simulink model "Subsystem"  (R2020b)
settings: Solver=VariableStepAuto  StartTime=0.0  StopTime=10.0  RelTol=1e-3
settings Model: Creator=shivanshu shukla  LastModifiedBy=shivanshu shukla
settings DataIOCC: SaveOutput=off  SaveTime=off

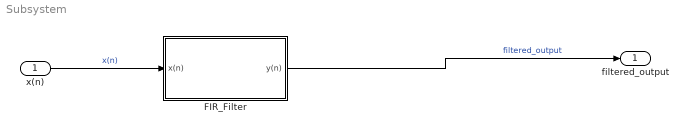
== system Subsystem ==
  x(n) : Inport  OutDataTypeStr=double  PortDimensions=1  SampleTime=[0,1]
  FIR_Filter : Subsystem  TreatAsAtomicUnit=on
  filtered_output : Outport  OutDataTypeStr=double  PortDimensions=1  SampleTime=[0,1]
  wires:
  x(n)/1 -> FIR_Filter/1(x(n))  "x(n)"
  FIR_Filter/1(y(n)) -> filtered_output/1  "filtered_output"

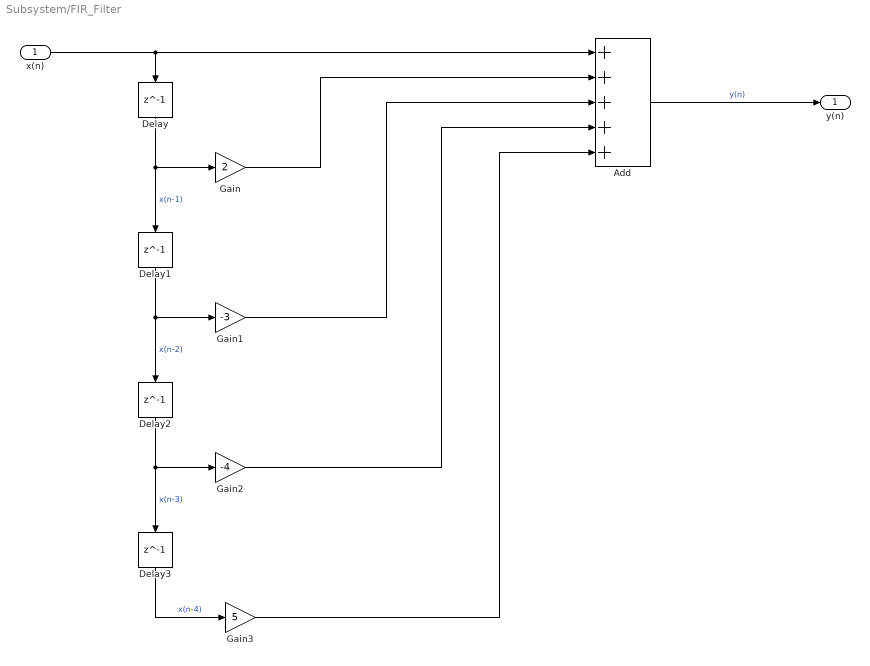
== system Subsystem/FIR_Filter ==
  x(n) : Inport
  Add : Sum  Inputs=+++++
  Delay{,1..3} (4 alike) : Delay  DelayLength=1
  Gain : Gain  Gain=2
  Gain1 : Gain  Gain=-3
  Gain2 : Gain  Gain=-4
  Gain3 : Gain  Gain=5
  y(n) : Outport
  wires:
  Add/1 -> y(n)/1  "y(n)"
  Gain3/1 -> Add/5
  Delay3/1 -> Gain3/1  "x(n-4)"
  Gain1/1 -> Add/3
  x(n)/1 -> Add/1, Delay/1
  Delay2/1 -> Delay3/1, Gain2/1  "x(n-3)"
  Gain/1 -> Add/2
  Delay1/1 -> Delay2/1, Gain1/1  "x(n-2)"
  Gain2/1 -> Add/4
  Delay/1 -> Delay1/1, Gain/1  "x(n-1)"
